simulink library "Lib_PFSys_GenericGenerator_TMATS"  (R2019b)
settings: Solver=ode45  StartTime=0.0  StopTime=10.0  RelTol=1e-3  EnableMultiTasking=on
Description:
  | Thomas Modules
settings Model: Creator=jwchapm2  LastModifiedBy=mebell
settings DataIOCC: LimitDataPoints=on  SaveFormat=Array  ReturnWorkspaceOutputs=off
settings OptimizationCC: ExpressionDepthLimit=2147483647  LifeSpan=inf
settings DebuggingCC: UnderspecifiedInitializationDetection=Classic  MergeDetectMultiDrivingBlocksExec=none  SolverPrmCheckMsg=warning  StateNameClashWarn=warning  SFUnexpectedBacktrackingDiag=warning  SFNoUnconditionalDefaultTransitionDiag=warning  SFExecutionAtInitializationDiag=none  ArithmeticOperatorsInVariantConditions=warning
settings HardwareCC: ProdBitPerPointer=32  ProdBitPerSizeT=32  ProdBitPerPtrDiffT=32  ProdLargestAtomicFloat=None  ProdIntDivRoundTo=Undefined  ProdEndianess=Unspecified  ProdWordSize=32  ProdHWDeviceType=32-bit Generic
settings ModelReferenceCC: PropagateSignalLabelsOutOfModel=off
settings SFSimCC: SimUseLocalCustomCode=off  CustomCodeUndefinedFunction=UseInterfaceOnly
settings RTWCC: RTWUseLocalCustomCode=off
settings CodeAppCC: StateflowObjectComments=on
settings GRTTargetCC: TargetLangStandard=C89/C90 (ANSI)  GeneratePreprocessorConditionals=Disable all
settings ConfigComp: CovMetricSettings=dw  CovHtmlReporting=on  CovSaveCumulativeToWorkspaceVar=on  CovSaveSingleToWorkspaceVar=on  CovExternalEMLEnable=off

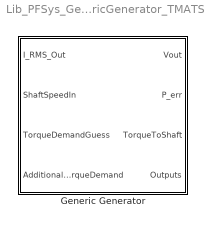
== system Lib_PFSys_GenericGenerator_TMATS ==
  Generic Generator : Subsystem  mask(Motor){X_C_SpeedVec_M=[0.0 0.1 1.0], Y_C_TorqueVec_M=[0.0 0.1 1.0], T_C_EffArray_M=[0.5 0.5 0.5; 0.5 1.0 1.0; 0.5 1.0 1.0], Ke_M=0.5}
      mask prompts: X_C_SpeedVec_M "X_C_SpeedVec_M - Efficiency Table Speed Vector (X-axis)(nx1)"; Y_C_TorqueVec_M "Y_C_TorqueVec_M - Efficiency Table Torque Vector (Y-axis)(mx1)"; T_C_EffArray_M "T_C_EffArray_M - Efficiency Table Values (Eff = f(i, V)(nxm)"; Ke_M "Ke_M - Motor EMF Constant (V/ rad/s)"
      mask help:
      | This block represents a generic motor with a purely resistive input
      | impedance, and a lumped efficiency/loss model, specified as a lookup table.

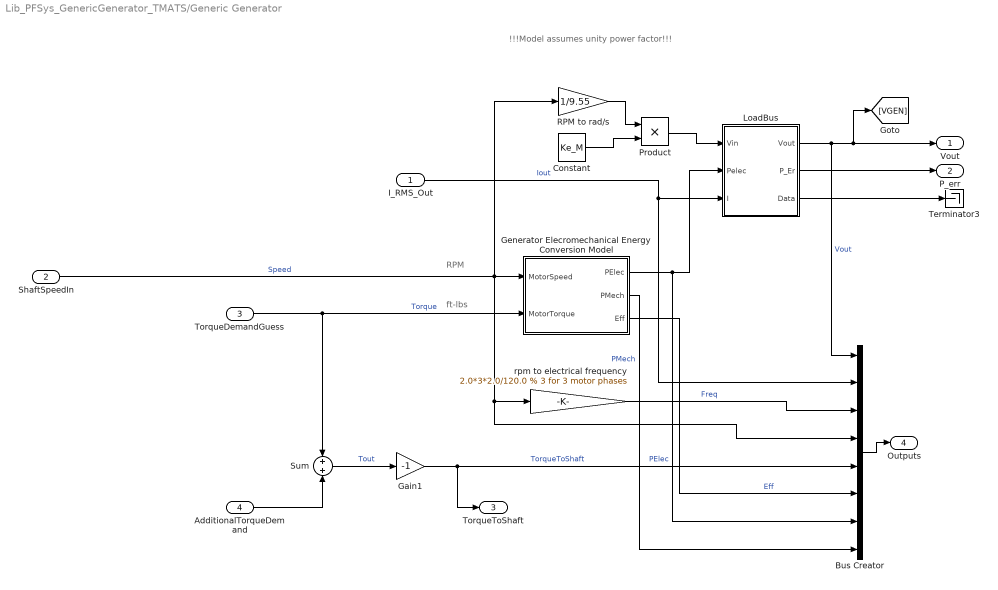
== system Lib_PFSys_GenericGenerator_TMATS/Generic Generator ==
  note: ft-lbs
  note: RPM
  note: !!!Model assumes unity power factor!!!
  I_RMS_Out : Inport
  ShaftSpeedIn : Inport  Port=2
  TorqueDemandGuess : Inport  Port=3
  AdditionalTorqueDemand : Inport  Port=4
  Bus Creator : BusCreator  Inputs=8
  Constant : Constant  Value=Ke_M
  Gain1 : Gain  Gain=-1
  Generator Elecromechanical Energy Conversion Model : Subsystem
  LoadBus : Subsystem  AncestorBlock=Lib_PF_BusLoadDC_TMATS/LoadBus DC  mask{PeInEN_M=on, P_M=-2, BlkNm_M=double(gcb)}
      mask prompts: PeInEN_M "PeInEN_M - External Pelec"; P_M "P_M - Real power"; BlkNm_M "Block name as double for simulink output"
      mask init:
      | %Manage Power Inputs
      | if PeInEN_M == 1
      |     if strcmp(get_param([BlkNm_M '/Pelec'],'BlockType'),'Constant')
      |         MSK_ReplaceBlock_TMATS([BlkNm_M '/Pelec'],'built-in/Inport');
      |     end
      |     set_param([BlkNm_M '/Pelec'],'Port',num2str(2));
      | elseif PeInEN_M == 0
      |     if strcmp(get_param([BlkNm_M '/Pelec'],'BlockType'),'Inport')
      |         MSK_ReplaceBlock_TMATS([BlkNm_M '/Pelec'],'built-in/Constant');
      |         set_param([BlkNm_M '/Pelec'],'Value','P_M');
      |     end
      | end
      mask Callback PeInEN_M: MSK_SEC_Enables_TMATS('PeInEN_M',2,'dis')
  Product : Product
  RPM to rad/s : Gain  Gain=1/9.55
  Sum : Sum
  Terminator3 : Terminator
  rpm to electrical frequency : Gain  Gain=2.0*3*2.0/120.0 % 3 for 3 motor phases
  Vout : Outport
  P_err : Outport  Port=2  VectorParamsAs1DForOutWhenUnconnected=off
  TorqueToShaft : Outport  Port=3
  Outputs : Outport  Port=4  VectorParamsAs1DForOutWhenUnconnected=off
  wires:
  Generator Elecromechanical Energy Conversion Model/1(PElec) -> Bus Creator/7, LoadBus/2(Pelec)  "PElec"
  Bus Creator/1 -> Outputs/1
  rpm to electrical frequency/1 -> Bus Creator/3  "Freq"
  TorqueDemandGuess/1 -> Sum/1, Generator Elecromechanical Energy Conversion Model/2(MotorTorque)  "Torque"
  ShaftSpeedIn/1 -> RPM to rad/s/1, Generator Elecromechanical Energy Conversion Model/1(MotorSpeed), Bus Creator/4, rpm to electrical frequency/1  "Speed"
  LoadBus/3(Data) -> Terminator3/1
  LoadBus/2(P_Er) -> P_err/1
  LoadBus/1(Vout) -> [VGEN], Vout/1, Bus Creator/1  "Vout"
  Generator Elecromechanical Energy Conversion Model/3(Eff) -> Bus Creator/6  "Eff"
  Generator Elecromechanical Energy Conversion Model/2(PMech) -> Bus Creator/8  "PMech"
  Product/1 -> LoadBus/1(Vin)
  RPM to rad/s/1 -> Product/1
  Constant/1 -> Product/2
  Gain1/1 -> Bus Creator/5, TorqueToShaft/1  "TorqueToShaft"
  I_RMS_Out/1 -> Bus Creator/2, LoadBus/3(I)  "Iout"
  AdditionalTorqueDemand/1 -> Sum/2
  Sum/1 -> Gain1/1  "Tout"

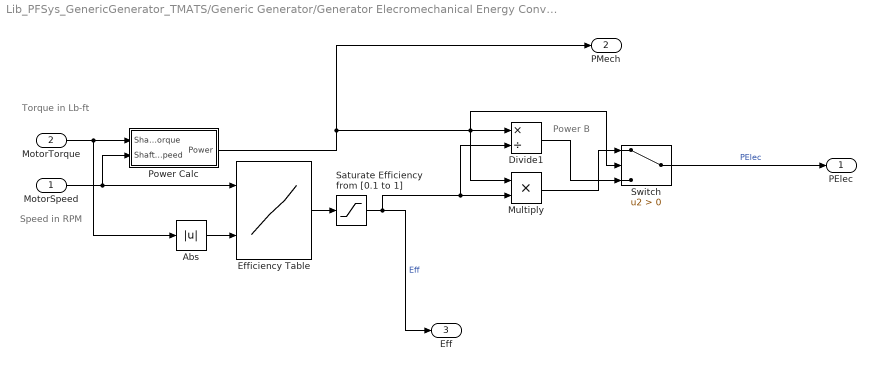
== system Lib_PFSys_GenericGenerator_TMATS/Generic Generator/Generator Elecromechanical Energy Conversion Model ==
  note: Speed in RPM
  note: Torque in Lb-ft
  note: Power B
  MotorSpeed : Inport
  MotorTorque : Inport  Port=2
  Abs : Abs
  Divide1 : Product  Inputs=*/
  Efficiency Table : Lookup_n-D  BreakpointsForDimension1=X_C_SpeedVec_M  BreakpointsForDimension2=Y_C_TorqueVec_M  Table=T_C_EffArray_M  ExtrapMethod=Clip  InternalRulePriority=Speed  RndMeth=Simplest  InputSameDT=on
  Multiply : Product
  Power Calc : Subsystem
  Saturate Efficiency from [0.1 to 1] : Saturate  UpperLimit=1  LowerLimit=0.1
  Switch : Switch  Criteria=u2 > Threshold
  PElec : Outport  VectorParamsAs1DForOutWhenUnconnected=off
  PMech : Outport  Port=2  VectorParamsAs1DForOutWhenUnconnected=off
  Eff : Outport  Port=3  VectorParamsAs1DForOutWhenUnconnected=off
  wires:
  Efficiency Table/1 -> Saturate Efficiency from [0.1 to 1]/1
  Saturate Efficiency from [0.1 to 1]/1 -> Divide1/2, Multiply/2, Eff/1  "Eff"
  Abs/1 -> Efficiency Table/2
  Switch/1 -> PElec/1  "PElec"
  MotorTorque/1 -> Abs/1, Power Calc/1(ShaftTorque)
  MotorSpeed/1 -> Power Calc/2(ShaftSpeed), Efficiency Table/1
  Divide1/1 -> Switch/3
  Multiply/1 -> Switch/1
  Power Calc/1(Power) -> Switch/2, Multiply/1, Divide1/1, PMech/1

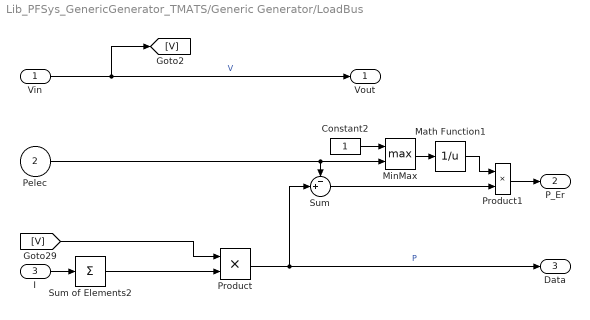
== system Lib_PFSys_GenericGenerator_TMATS/Generic Generator/LoadBus ==
  Vin : Inport
  Pelec : Inport  Port=2
  I : Inport  Port=3
  Constant2 : Constant
  Math Function1 : Math  Operator=reciprocal  SaturateOnIntegerOverflow=on
  MinMax : MinMax  Function=max  Inputs=2
  Product : Product
  Product1 : Product
  Sum : Sum  Inputs=-+|
  Sum of Elements2 : Sum  Inputs=+
  Vout : Outport
  P_Er : Outport  Port=2
  Data : Outport  Port=3
  wires:
  Sum/1 -> Product1/2
  Product1/1 -> P_Er/1
  Math Function1/1 -> Product1/1
  MinMax/1 -> Math Function1/1
  Constant2/1 -> MinMax/1
  Pelec/1 -> Sum/1, MinMax/2
  Vin/1 -> [V], Vout/1  "V"
  Product/1 -> Sum/2, Data/1  "P"
  I/1 -> Sum of Elements2/1
  [V] -> Product/1
  Sum of Elements2/1 -> Product/2

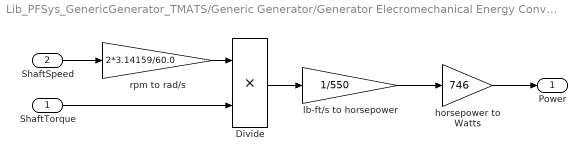
== system Lib_PFSys_GenericGenerator_TMATS/Generic Generator/Generator Elecromechanical Energy Conversion Model/Power Calc ==
  ShaftTorque : Inport
  ShaftSpeed : Inport  Port=2
  Divide : Product  Inputs=**
  horsepower to Watts : Gain  Gain=746
  lb-ft/s to horsepower : Gain  Gain=1/550
  rpm to rad/s : Gain  Gain=2*3.14159/60.0
  Power : Outport  VectorParamsAs1DForOutWhenUnconnected=off
  wires:
  ShaftSpeed/1 -> rpm to rad/s/1
  Divide/1 -> lb-ft/s to horsepower/1
  lb-ft/s to horsepower/1 -> horsepower to Watts/1
  ShaftTorque/1 -> Divide/2
  rpm to rad/s/1 -> Divide/1
  horsepower to Watts/1 -> Power/1
